simulink model "case_1"  (R2022a)
settings: Solver=VariableStepAuto  StartTime=0.0  StopTime=50  RelTol=1e-3
undefined symbols (not defined in the file): c, m
settings Model: Creator=Z0150218  LastModifiedBy=Z0150218

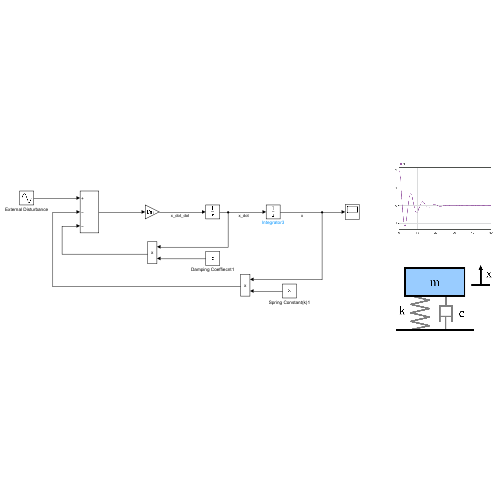
[thumbnail: Simulink's stored preview of the top-level diagram]
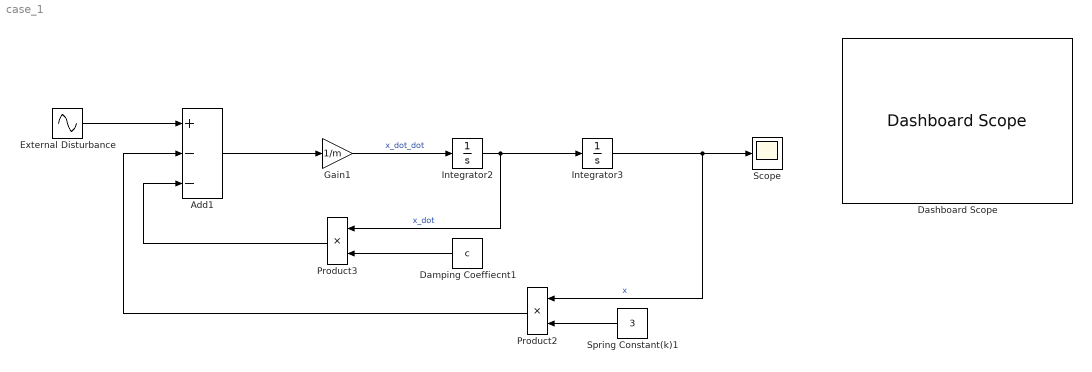
== system case_1 ==
  Add1 : Sum  Inputs=+--
  Damping Coeffiecnt1 : Constant  Value=c
  Dashboard Scope : DashboardScope
  External Disturbance : Sin  Amplitude=0.01  SampleTime=0
  Gain1 : Gain  Gain=1/m
  Integrator2 : Integrator
  Integrator3 : Integrator  InitialCondition=2
  Product2 : Product
  Product3 : Product
  Scope : Scope
  Spring Constant(k)1 : Constant  Value=3
  wires:
  Integrator2/1 -> Product3/1, Integrator3/1  "x_dot"
  Gain1/1 -> Integrator2/1  "x_dot_dot"
  Integrator3/1 -> Scope/1, Product2/1  "x"
  Add1/1 -> Gain1/1
  Spring Constant(k)1/1 -> Product2/2
  Product2/1 -> Add1/2
  Damping Coeffiecnt1/1 -> Product3/2
  Product3/1 -> Add1/3
  External Disturbance/1 -> Add1/1
